simulink model "thirdweek_third"  (R2020a)
settings: Solver=VariableStepAuto  StartTime=0.0  StopTime=10.0  RelTol=1e-3
model workspace (MAT data in the model file):
  Kd = Simulink.Parameter
  Kd.Value = 50
  Kd.DataType = 'auto'
  Kd.Dimensions = [1 1]
  Ki = Simulink.Parameter
  Ki.Value = 300
  Ki.DataType = 'auto'
  Ki.Dimensions = [1 1]
  Kp = Simulink.Parameter
  Kp.Value = 350
  Kp.DataType = 'auto'
  Kp.Dimensions = [1 1]
settings Model: Creator=Admin  LastModifiedBy=Admin

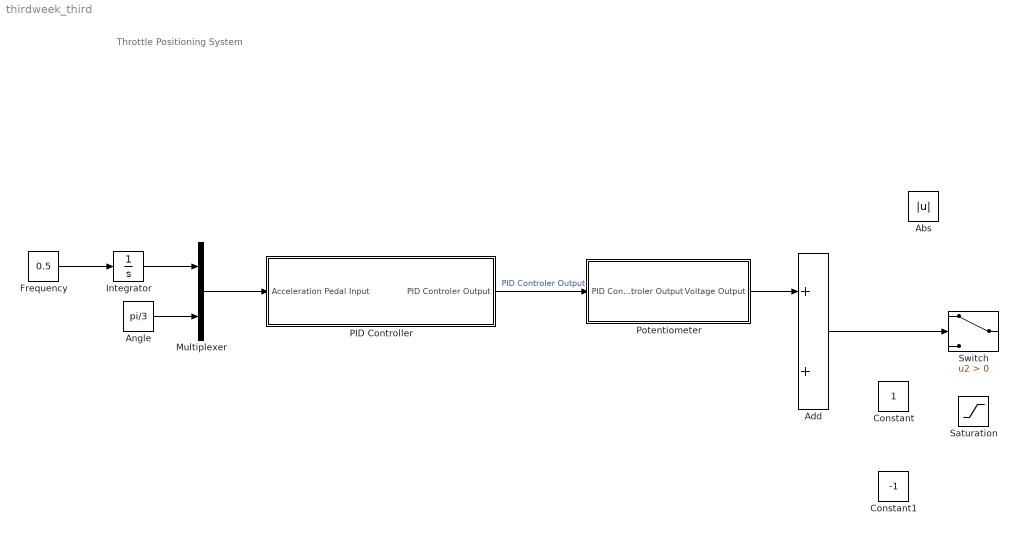
== system thirdweek_third ==
  note: Throttle Positioning System
  Abs : Abs
  Add : Sum
  Angle : Constant  Value=pi/3
  Constant : Constant
  Constant1 : Constant  Value=-1
  Frequency : Constant  Value=0.5
  Integrator : Integrator
  Multiplexer : Mux  Inputs=2
  PID Controller : Subsystem
  Potentiometer : Subsystem
  Saturation : Saturate
  Switch : Switch  Criteria=u2 > Threshold
  wires:
  Frequency/1 -> Integrator/1
  Integrator/1 -> Multiplexer/1
  Angle/1 -> Multiplexer/2
  Multiplexer/1 -> PID Controller/1(Acceleration Pedal Input)
  PID Controller/1(PID Controler Output) -> Potentiometer/1(PID Controler Output)  "PID Controler Output"
  Potentiometer/1(Voltage Output) -> Add/1
  Add/1 -> Switch/2

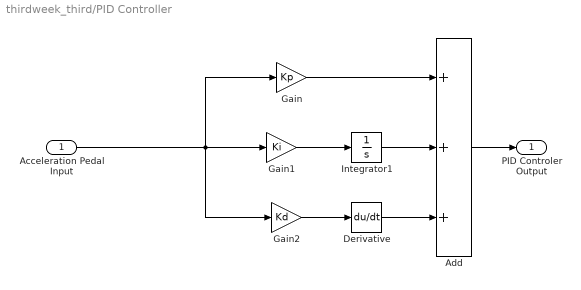
== system thirdweek_third/PID Controller ==
  Acceleration Pedal Input : Inport
  Add : Sum  Inputs=+++
  Derivative : Derivative
  Gain : Gain  Gain=Kp
  Gain1 : Gain  Gain=Ki
  Gain2 : Gain  Gain=Kd
  Integrator1 : Integrator
  PID Controler Output : Outport
  wires:
  Add/1 -> PID Controler Output/1
  Derivative/1 -> Add/3
  Gain/1 -> Add/1
  Integrator1/1 -> Add/2
  Gain1/1 -> Integrator1/1
  Acceleration Pedal Input/1 -> Gain2/1, Gain/1, Gain1/1
  Gain2/1 -> Derivative/1

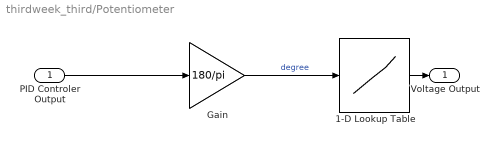
== system thirdweek_third/Potentiometer ==
  PID Controler Output : Inport
  1-D Lookup Table : Lookup_n-D  NumberOfTableDimensions=1  BreakpointsForDimension1=[0 90]  Table=[0.5 0.45]  InternalRulePriority=Speed  RndMeth=Simplest  InputSameDT=on
  Gain : Gain  Gain=180/pi
  Voltage Output : Outport
  wires:
  Gain/1 -> 1-D Lookup Table/1  "degree"
  1-D Lookup Table/1 -> Voltage Output/1
  PID Controler Output/1 -> Gain/1
